simulink model "CL_CC"  (R2015b)
settings: Solver=FixedStepDiscrete  StartTime=0.0  StopTime=final_time  RelTol=1e-3
undefined symbols (not defined in the file): BMSk_stepSize, cell_ocvs_sampling, cell_socs_sampling, cell_temps_sampling, cell_voltages_sampling, charge_cycle, inital_outlet_temperature, initial_cell_ocvs, initial_cell_socs, initial_cell_temps, initial_cell_voltages, initial_pack_current, initial_pack_soc, initial_pack_voltage, initial_vehicle_side_voltage, pack_current_sampling, pack_soc_sampling, pack_voltage_sampling, sigbuilder_block, vehicle_side_voltage_sampling
libraries: simulink x5
(part 2 of 2)

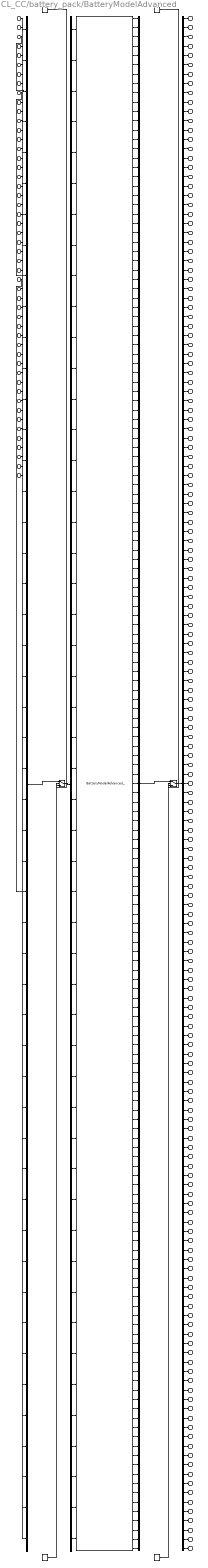
== system CL_CC/battery_pack/BatteryModelAdvanced ==
  cmd_1 : Inport
  cmd_2 : Inport  Port=2
  cmd_3 : Inport  Port=3
  cmd_4 : Inport  Port=4
  cmd_5 : Inport  Port=5
  cmd_6 : Inport  Port=6
  cmd_7 : Inport  Port=7
  cmd_8 : Inport  Port=8
  cmd_9 : Inport  Port=9
  cmd_10 : Inport  Port=10
  cmd_11 : Inport  Port=11
  cmd_12 : Inport  Port=12
  cmd_13 : Inport  Port=13
  cmd_14 : Inport  Port=14
  cmd_15 : Inport  Port=15
  cmd_16 : Inport  Port=16
  cmd_17 : Inport  Port=17
  cmd_18 : Inport  Port=18
  cmd_19 : Inport  Port=19
  cmd_20 : Inport  Port=20
  cmd_21 : Inport  Port=21
  cmd_22 : Inport  Port=22
  cmd_23 : Inport  Port=23
  cmd_24 : Inport  Port=24
  cmd_25 : Inport  Port=25
  cmd_26 : Inport  Port=26
  cmd_27 : Inport  Port=27
  cmd_28 : Inport  Port=28
  cmd_29 : Inport  Port=29
  cmd_30 : Inport  Port=30
  cmd_31 : Inport  Port=31
  cmd_32 : Inport  Port=32
  cmd_33 : Inport  Port=33
  cmd_34 : Inport  Port=34
  cmd_35 : Inport  Port=35
  cmd_36 : Inport  Port=36
  cmd_37 : Inport  Port=37
  cmd_38 : Inport  Port=38
  cmd_39 : Inport  Port=39
  cmd_40 : Inport  Port=40
  main_cc_comd : Inport  Port=41
  pre_cc_cmd : Inport  Port=42
  neg_cc_cmd : Inport  Port=43
  chg_cc_cmd : Inport  Port=44
  fan_cmd : Inport  Port=45
  cabin_temp : Inport  Port=46
  Ichg_max : Inport  Port=47
  Idischg_max : Inport  Port=48
  input_current : Inport  Port=49
  load_type : Inport  Port=50
  Cmd_In : Constant  Value=[1 1 1 1 1 1 1 1 1 1 1 1 1 1 1 1 1 1 1 1 1 1 1 1 1 1 1 1 1 1 1 1 1 1 1 1 1 1 1 1 1 1 1 1 1 1 1 1 1 1]
  Cmd_Out : Constant  Value=[1 1 1 1 1 1 1 1 1 1 1 1 1 1 1 1 1 1 1 1 1 1 1 1 1 1 1 1 1 1 1 1 1 1 1 1 1 1 1 1 1 1 1 1 1 1 1 1 1 1 1 1 1 1 1 1 1 1 1 1 1 1 1 1 1 1 1 1 1 1 1 1 1 1 1 1 1 1 1 1 1 1 1 1 1 1 1 1 1 1 1 1 1 1 1 1 1 1 1 1 1 1 1 1 1 1 1 1 1 1 1 1 1 1 1 1 1 1 1 1 1 1 1 1 1 1 1 1 1 1 1 1 1 1 1 1 1 1 1 1 1 1 1 1 1 1 1 1 1 1 1 1 1 1 1 1 1 1 1 1 1 1 1 1 1]
  Constant_In : Constant  Value=[0 0 0 0 0 0 0 0 0 0 0 0 0 0 0 0 0 0 0 0 0 0 0 0 0 0 0 0 0 0 0 0 0 0 0 0 0 0 0 0 0 0 0 0 0 0 0 0 0 0]
  Constant_Out : Constant  Value=[0 0 0 0 0 0 0 0 0 0 0 0 0 0 0 0 0 0 0 0 0 0 0 0 0 0 0 0 0 0 0 0 0 0 0 0 0 0 0 0 0 0 0 0 0 0 0 0 0 0 0 0 0 0 0 0 0 0 0 0 0 0 0 0 0 0 0 0 0 0 0 0 0 0 0 0 0 0 0 0 0 0 0 0 0 0 0 0 0 0 0 0 0 0 0 0 0 0 0 0 0 0 0 0 0 0 0 0 0 0 0 0 0 0 0 0 0 0 0 0 0 0 0 0 0 0 0 0 0 0 0 0 0 0 0 0 0 0 0 0 0 0 0 0 0 0 0 0 0 0 0 0 0 0 0 0 0 0 0 0 0 0 0 0 0]
  Demux_In : Demux  Outputs=50
  Demux_Out : Demux  Outputs=165
  Mux_In : Mux  Inputs=50
  Mux_Out : Mux  Inputs=165
  S-Function : S-Function  InitFcn=clear BatteryModelAdvanced_  StopFcn=clear BatteryModelAdvanced_  FunctionName=BatteryModelAdvanced_  Parameters="[0.1;0.1;1e-06;0.1;100;0;0;2;0;1;0.001;0;1] ['tcase             ';'dcell             ';'Lcell             ';'Rcell             ';'Dcell2cell        ';'Tair              ';'cell_capacity     ';'initial_sohc      ';'initial_sohr      ';'balance_resistor  ';'Initial_SOC       ';'imbalance_cell_soc';'load_cycle_type   '] [5;2.009e-06;206;37;77;35;8;100;100;1;60;60;1] [] [] ['cycle_name'] ['Drive_Cycles/FTP_72.data']"  SFunctionDeploymentMode=off  EnableBusSupport=off
      mask Display: port_label('output',1,'Cell_Voltage1');port_label('output',2,'Cell_Voltage2');port_label('output',3,'Cell_Voltage3');port_label('output',4,'Cell_Voltage4');port_label('output',5,'Cell_Voltage5');port_label('output',6,'Cell_Voltage6');port_label('output',7,'Cell_Voltage7');port_label('output',8,'Cell_Voltage8');port_label('output',9,'Cell_Voltage9');port_label('output',10,'Cell_Voltage10');port_label('output',11,'Cell_Voltage11');port_label('output',12,'Cell_Voltage12');port_label('output',13,'Cell_Voltage13');port_label('output',14,'Cell_Voltage14');port_label('output',15,'Cell_Voltage15');port_label('output',16,'Cell_Voltage16');port_label('output',17,'Cell_Voltage17');port_label('output',18,'Cell_Voltage18');port_label('output',19,'Cell_Voltage19');port_label('output',20,'Cell_Voltage20');port_label('output',21,'Cell_Voltage21');port_label('output',22,'Cell_Voltage22');port_label('output',23,'Cell_Voltage23');port_label('output',24,'Cell_Voltage24');port_label('output',25,'Cell_Voltage25');port_label('output',26,'Cell_Voltage26');port_label('output',27,'Cell_Voltage27');port_label('output',28,'Cell_Voltage28');port_label('output',29,'Cell_Voltage29');port_label('output',30,'Cell_Voltage30');port_label('output',31,'Cell_Voltage31');port_label('output',32,'Cell_Voltage32');port_label('output',33,'Cell_Voltage33');port_label('output',34,'Cell_Voltage34');port_label('output',35,'Cell_Voltage35');port_label('output',36,'Cell_Voltage36');port_label('output',37,'Cell_Voltage37');port_label('output',38,'Cell_Voltage38');port_label('output',39,'Cell_Voltage39');port_label('output',40,'Cell_Voltage40');port_label('output',41,'Cell_temp1');port_label('output',42,'Cell_temp2');port_label('output',43,'Cell_temp3');port_label('output',44,'Cell_temp4');port_label('output',45,'Cell_temp5');port_label('output',46,'Cell_temp6');port_label('output',47,'Cell_temp7');port_label('output',48,'Cell_temp8');port_label('output',49,'Cell_temp9');port_label('output',50,'Cell_temp10');port_label('output',51,'Cell_temp11');port_label('output',52,'Cell_temp12');port_label('output',53,'Cell_temp13');port_label('output',54,'Cell_temp14');port_label('output',55,'Cell_temp15');port_label('output',56,'Cell_temp16');port_label('output',57,'Cell_temp17');port_label('output',58,'Cell_temp18');port_label('output',59,'Cell_temp19');port_label('output',60,'Cell_temp20');port_label('output',61,'Cell_temp21');port_label('output',62,'Cell_temp22');port_label('output',63,'Cell_temp23');port_label('output',64,'Cell_temp24');port_label('output',65,'Cell_temp25');port_label('output',66,'Cell_temp26');port_label('output',67,'Cell_temp27');port_label('output',68,'Cell_temp28');port_label('output',69,'Cell_temp29');port_label('output',70,'Cell_temp30');port_label('output',71,'Cell_temp31');port_label('output',72,'Cell_temp32');port_label('output',73,'Cell_temp33');port_label('output',74,'Cell_temp34');port_label('output',75,'Cell_temp35');port_label('output',76,'Cell_temp36');port_label('output',77,'Cell_temp37');port_label('output',78,'Cell_temp38');port_label('output',79,'Cell_temp39');port_label('output',80,'Cell_temp40');port_label('output',81,'Cell_soc1');port_label('output',82,'Cell_soc2');port_label('output',83,'Cell_soc3');port_label('output',84,'Cell_soc4');port_label('output',85,'Cell_soc5');port_label('output',86,'Cell_soc6');port_label('output',87,'Cell_soc7');port_label('output',88,'Cell_soc8');port_label('output',89,'Cell_soc9');port_label('output',90,'Cell_soc10');port_label('output',91,'Cell_soc11');port_label('output',92,'Cell_soc12');port_label('output',93,'Cell_soc13');port_label('output',94,'Cell_soc14');port_label('output',95,'Cell_soc15');port_label('output',96,'Cell_soc16');port_label('output',97,'Cell_soc17');port_label('output',98,'Cell_soc18');port_label('output',99,'Cell_soc19');port_label('output',100,'Cell_soc20');port_label('output',101,'Cell_soc21');port_label('output',102,'Cell_soc22');port_label('output',103,'Cell_soc23');port_label('output',104,'Cell_soc24');port_label('output',105,'Cell_soc25');port_label('output',106,'Cell_soc26');port_label('output',107,'Cell_soc27');port_label('output',108,'Cell_soc28');port_label('output',109,'Cell_soc29');port_label('output',110,'Cell_soc30');port_label('output',111,'Cell_soc31');port_label('output',112,'Cell_soc32');port_label('output',113,'Cell_soc33');port_label('output',114,'Cell_soc34');port_label('output',115,'Cell_soc35');port_label('output',116,'Cell_soc36');port_label('output',117,'Cell_soc37');port_label('output',118,'Cell_soc38');port_label('output',119,'Cell_soc39');port_label('output',120,'Cell_soc40');port_label('output',121,'Cell_ocv1');port_label('output',122,'Cell_ocv2');port_label('output',123,'Cell_ocv3');port_label('output',124,'Cell_ocv4');port_label('output',125,'Cell_ocv5');port_label('output',126,'Cell_ocv6');port_label('output',127,'Cell_ocv7');port_label('output',128,'Cell_ocv8');port_label('output',129,'Cell_ocv9');port_label('output',130,'Cell_ocv10');port_label('output',131,'Cell_ocv11');port_label('output',132,'Cell_ocv12');port_label('output',133,'Cell_ocv13');port_label('output',134,'Cell_ocv14');port_label('output',135,'Cell_ocv15');port_label('output',136,'Cell_ocv16');port_label('output',137,'Cell_ocv17');port_label('output',138,'Cell_ocv18');port_label('output',139,'Cell_ocv19');port_label('output',140,'Cell_ocv20');port_label('output',141,'Cell_ocv21');port_label('output',142,'Cell_ocv22');port_label('output',143,'Cell_ocv23');port_label('output',144,'Cell_ocv24');port_label('output',145,'Cell_ocv25');port_label('output',146,'Cell_ocv26');port_label('output',147,'Cell_ocv27');port_label('output',148,'Cell_ocv28');port_label('output',149,'Cell_ocv29');port_label('output',150,'Cell_ocv30');port_label('output',151,'Cell_ocv31');port_label('output',152,'Cell_ocv32');port_label('output',153,'Cell_ocv33');port_label('output',154,'Cell_ocv34');port_label('output',155,'Cell_ocv35');port_label('output',156,'Cell_ocv36');port_label('output',157,'Cell_ocv37');port_label('output',158,'Cell_ocv38');port_label('output',159,'Cell_ocv39');port_label('output',160,'Cell_ocv40');port_label('output',161,'outlet_temperature');port_label('output',162,'pack_voltage');port_label('output',163,'vehicle_side_voltage');port_label('output',164,'pack_current');port_label('output',165,'pack_soc');port_label('input',1,'cmd_1');port_label('input',2,'cmd_2');port_label('input',3,'cmd_3');port_label('input',4,'cmd_4');port_label('input',5,'cmd_5');port_label('input',6,'cmd_6');port_label('input',7,'cmd_7');port_label('input',8,'cmd_8');port_label('input',9,'cmd_9');port_label('input',10,'cmd_10');port_label('input',11,'cmd_11');port_label('input',12,'cmd_12');port_label('input',13,'cmd_13');port_label('input',14,'cmd_14');port_label('input',15,'cmd_15');port_label('input',16,'cmd_16');port_label('input',17,'cmd_17');port_label('input',18,'cmd_18');port_label('input',19,'cmd_19');port_label('input',20,'cmd_20');port_label('input',21,'cmd_21');port_label('input',22,'cmd_22');port_label('input',23,'cmd_23');port_label('input',24,'cmd_24');port_label('input',25,'cmd_25');port_label('input',26,'cmd_26');port_label('input',27,'cmd_27');port_label('input',28,'cmd_28');port_label('input',29,'cmd_29');port_label('input',30,'cmd_30');port_label('input',31,'cmd_31');port_label('input',32,'cmd_32');port_label('input',33,'cmd_33');port_label('input',34,'cmd_34');port_label('input',35,'cmd_35');port_label('input',36,'cmd_36');port_label('input',37,'cmd_37');port_label('input',38,'cmd_38');port_label('input',39,'cmd_39');port_label('input',40,'cmd_40');port_label('input',41,'main_cc_comd');port_label('input',42,'pre_cc_cmd');port_label('input',43,'neg_cc_cmd');port_label('input',44,'chg_cc_cmd');port_label('input',45,'fan_cmd');port_label('input',46,'cabin_temp');port_label('input',47,'Ichg_max');port_label('input',48,'Idischg_max');port_label('input',49,'input_current');port_label('input',50,'load_type');disp('Simcenter Amesim:\n BatteryModelAdvanced_')
  Switch_In : Switch  Threshold=0.5  SaturateOnIntegerOverflow=on  InputSameDT=on
  Switch_Out : Switch  Threshold=0.5  SaturateOnIntegerOverflow=on  InputSameDT=on
  Cell_Voltage1 : Outport
  Cell_Voltage2 : Outport  Port=2
  Cell_Voltage3 : Outport  Port=3
  Cell_Voltage4 : Outport  Port=4
  Cell_Voltage5 : Outport  Port=5
  Cell_Voltage6 : Outport  Port=6
  Cell_Voltage7 : Outport  Port=7
  Cell_Voltage8 : Outport  Port=8
  Cell_Voltage9 : Outport  Port=9
  Cell_Voltage10 : Outport  Port=10
  Cell_Voltage11 : Outport  Port=11
  Cell_Voltage12 : Outport  Port=12
  Cell_Voltage13 : Outport  Port=13
  Cell_Voltage14 : Outport  Port=14
  Cell_Voltage15 : Outport  Port=15
  Cell_Voltage16 : Outport  Port=16
  Cell_Voltage17 : Outport  Port=17
  Cell_Voltage18 : Outport  Port=18
  Cell_Voltage19 : Outport  Port=19
  Cell_Voltage20 : Outport  Port=20
  Cell_Voltage21 : Outport  Port=21
  Cell_Voltage22 : Outport  Port=22
  Cell_Voltage23 : Outport  Port=23
  Cell_Voltage24 : Outport  Port=24
  Cell_Voltage25 : Outport  Port=25
  Cell_Voltage26 : Outport  Port=26
  Cell_Voltage27 : Outport  Port=27
  Cell_Voltage28 : Outport  Port=28
  Cell_Voltage29 : Outport  Port=29
  Cell_Voltage30 : Outport  Port=30
  Cell_Voltage31 : Outport  Port=31
  Cell_Voltage32 : Outport  Port=32
  Cell_Voltage33 : Outport  Port=33
  Cell_Voltage34 : Outport  Port=34
  Cell_Voltage35 : Outport  Port=35
  Cell_Voltage36 : Outport  Port=36
  Cell_Voltage37 : Outport  Port=37
  Cell_Voltage38 : Outport  Port=38
  Cell_Voltage39 : Outport  Port=39
  Cell_Voltage40 : Outport  Port=40
  Cell_temp1 : Outport  Port=41
  Cell_temp2 : Outport  Port=42
  Cell_temp3 : Outport  Port=43
  Cell_temp4 : Outport  Port=44
  Cell_temp5 : Outport  Port=45
  Cell_temp6 : Outport  Port=46
  Cell_temp7 : Outport  Port=47
  Cell_temp8 : Outport  Port=48
  Cell_temp9 : Outport  Port=49
  Cell_temp10 : Outport  Port=50
  Cell_temp11 : Outport  Port=51
  Cell_temp12 : Outport  Port=52
  Cell_temp13 : Outport  Port=53
  Cell_temp14 : Outport  Port=54
  Cell_temp15 : Outport  Port=55
  Cell_temp16 : Outport  Port=56
  Cell_temp17 : Outport  Port=57
  Cell_temp18 : Outport  Port=58
  Cell_temp19 : Outport  Port=59
  Cell_temp20 : Outport  Port=60
  Cell_temp21 : Outport  Port=61
  Cell_temp22 : Outport  Port=62
  Cell_temp23 : Outport  Port=63
  Cell_temp24 : Outport  Port=64
  Cell_temp25 : Outport  Port=65
  Cell_temp26 : Outport  Port=66
  Cell_temp27 : Outport  Port=67
  Cell_temp28 : Outport  Port=68
  Cell_temp29 : Outport  Port=69
  Cell_temp30 : Outport  Port=70
  Cell_temp31 : Outport  Port=71
  Cell_temp32 : Outport  Port=72
  Cell_temp33 : Outport  Port=73
  Cell_temp34 : Outport  Port=74
  Cell_temp35 : Outport  Port=75
  Cell_temp36 : Outport  Port=76
  Cell_temp37 : Outport  Port=77
  Cell_temp38 : Outport  Port=78
  Cell_temp39 : Outport  Port=79
  Cell_temp40 : Outport  Port=80
  Cell_soc1 : Outport  Port=81
  Cell_soc2 : Outport  Port=82
  Cell_soc3 : Outport  Port=83
  Cell_soc4 : Outport  Port=84
  Cell_soc5 : Outport  Port=85
  Cell_soc6 : Outport  Port=86
  Cell_soc7 : Outport  Port=87
  Cell_soc8 : Outport  Port=88
  Cell_soc9 : Outport  Port=89
  Cell_soc10 : Outport  Port=90
  Cell_soc11 : Outport  Port=91
  Cell_soc12 : Outport  Port=92
  Cell_soc13 : Outport  Port=93
  Cell_soc14 : Outport  Port=94
  Cell_soc15 : Outport  Port=95
  Cell_soc16 : Outport  Port=96
  Cell_soc17 : Outport  Port=97
  Cell_soc18 : Outport  Port=98
  Cell_soc19 : Outport  Port=99
  Cell_soc20 : Outport  Port=100
  Cell_soc21 : Outport  Port=101
  Cell_soc22 : Outport  Port=102
  Cell_soc23 : Outport  Port=103
  Cell_soc24 : Outport  Port=104
  Cell_soc25 : Outport  Port=105
  Cell_soc26 : Outport  Port=106
  Cell_soc27 : Outport  Port=107
  Cell_soc28 : Outport  Port=108
  Cell_soc29 : Outport  Port=109
  Cell_soc30 : Outport  Port=110
  Cell_soc31 : Outport  Port=111
  Cell_soc32 : Outport  Port=112
  Cell_soc33 : Outport  Port=113
  Cell_soc34 : Outport  Port=114
  Cell_soc35 : Outport  Port=115
  Cell_soc36 : Outport  Port=116
  Cell_soc37 : Outport  Port=117
  Cell_soc38 : Outport  Port=118
  Cell_soc39 : Outport  Port=119
  Cell_soc40 : Outport  Port=120
  Cell_ocv1 : Outport  Port=121
  Cell_ocv2 : Outport  Port=122
  Cell_ocv3 : Outport  Port=123
  Cell_ocv4 : Outport  Port=124
  Cell_ocv5 : Outport  Port=125
  Cell_ocv6 : Outport  Port=126
  Cell_ocv7 : Outport  Port=127
  Cell_ocv8 : Outport  Port=128
  Cell_ocv9 : Outport  Port=129
  Cell_ocv10 : Outport  Port=130
  Cell_ocv11 : Outport  Port=131
  Cell_ocv12 : Outport  Port=132
  Cell_ocv13 : Outport  Port=133
  Cell_ocv14 : Outport  Port=134
  Cell_ocv15 : Outport  Port=135
  Cell_ocv16 : Outport  Port=136
  Cell_ocv17 : Outport  Port=137
  Cell_ocv18 : Outport  Port=138
  Cell_ocv19 : Outport  Port=139
  Cell_ocv20 : Outport  Port=140
  Cell_ocv21 : Outport  Port=141
  Cell_ocv22 : Outport  Port=142
  Cell_ocv23 : Outport  Port=143
  Cell_ocv24 : Outport  Port=144
  Cell_ocv25 : Outport  Port=145
  Cell_ocv26 : Outport  Port=146
  Cell_ocv27 : Outport  Port=147
  Cell_ocv28 : Outport  Port=148
  Cell_ocv29 : Outport  Port=149
  Cell_ocv30 : Outport  Port=150
  Cell_ocv31 : Outport  Port=151
  Cell_ocv32 : Outport  Port=152
  Cell_ocv33 : Outport  Port=153
  Cell_ocv34 : Outport  Port=154
  Cell_ocv35 : Outport  Port=155
  Cell_ocv36 : Outport  Port=156
  Cell_ocv37 : Outport  Port=157
  Cell_ocv38 : Outport  Port=158
  Cell_ocv39 : Outport  Port=159
  Cell_ocv40 : Outport  Port=160
  outlet_temperature : Outport  Port=161
  pack_voltage : Outport  Port=162
  vehicle_side_voltage : Outport  Port=163
  pack_current : Outport  Port=164
  pack_soc : Outport  Port=165
  wires:
  Mux_In/1 -> Switch_In/1
  Cmd_In/1 -> Switch_In/2
  Constant_In/1 -> Switch_In/3
  Switch_In/1 -> Demux_In/1
  Mux_Out/1 -> Switch_Out/1
  Cmd_Out/1 -> Switch_Out/2
  Constant_Out/1 -> Switch_Out/3
  Switch_Out/1 -> Demux_Out/1
  cmd_1/1 -> Mux_In/1
  Demux_In/1 -> S-Function/1
  cmd_2/1 -> Mux_In/2
  Demux_In/2 -> S-Function/2
  cmd_3/1 -> Mux_In/3
  Demux_In/3 -> S-Function/3
  cmd_4/1 -> Mux_In/4
  Demux_In/4 -> S-Function/4
  cmd_5/1 -> Mux_In/5
  Demux_In/5 -> S-Function/5
  cmd_6/1 -> Mux_In/6
  Demux_In/6 -> S-Function/6
  cmd_7/1 -> Mux_In/7
  Demux_In/7 -> S-Function/7
  cmd_8/1 -> Mux_In/8
  Demux_In/8 -> S-Function/8
  cmd_9/1 -> Mux_In/9
  Demux_In/9 -> S-Function/9
  cmd_10/1 -> Mux_In/10
  Demux_In/10 -> S-Function/10
  cmd_11/1 -> Mux_In/11
  Demux_In/11 -> S-Function/11
  cmd_12/1 -> Mux_In/12
  Demux_In/12 -> S-Function/12
  cmd_13/1 -> Mux_In/13
  Demux_In/13 -> S-Function/13
  cmd_14/1 -> Mux_In/14
  Demux_In/14 -> S-Function/14
  cmd_15/1 -> Mux_In/15
  Demux_In/15 -> S-Function/15
  cmd_16/1 -> Mux_In/16
  Demux_In/16 -> S-Function/16
  cmd_17/1 -> Mux_In/17
  Demux_In/17 -> S-Function/17
  cmd_18/1 -> Mux_In/18
  Demux_In/18 -> S-Function/18
  cmd_19/1 -> Mux_In/19
  Demux_In/19 -> S-Function/19
  cmd_20/1 -> Mux_In/20
  Demux_In/20 -> S-Function/20
  cmd_21/1 -> Mux_In/21
  Demux_In/21 -> S-Function/21
  cmd_22/1 -> Mux_In/22
  Demux_In/22 -> S-Function/22
  cmd_23/1 -> Mux_In/23
  Demux_In/23 -> S-Function/23
  cmd_24/1 -> Mux_In/24
  Demux_In/24 -> S-Function/24
  cmd_25/1 -> Mux_In/25
  Demux_In/25 -> S-Function/25
  cmd_26/1 -> Mux_In/26
  Demux_In/26 -> S-Function/26
  cmd_27/1 -> Mux_In/27
  Demux_In/27 -> S-Function/27
  cmd_28/1 -> Mux_In/28
  Demux_In/28 -> S-Function/28
  cmd_29/1 -> Mux_In/29
  Demux_In/29 -> S-Function/29
  cmd_30/1 -> Mux_In/30
  Demux_In/30 -> S-Function/30
  cmd_31/1 -> Mux_In/31
  Demux_In/31 -> S-Function/31
  cmd_32/1 -> Mux_In/32
  Demux_In/32 -> S-Function/32
  cmd_33/1 -> Mux_In/33
  Demux_In/33 -> S-Function/33
  cmd_34/1 -> Mux_In/34
  Demux_In/34 -> S-Function/34
  cmd_35/1 -> Mux_In/35
  Demux_In/35 -> S-Function/35
  cmd_36/1 -> Mux_In/36
  Demux_In/36 -> S-Function/36
  cmd_37/1 -> Mux_In/37
  Demux_In/37 -> S-Function/37
  cmd_38/1 -> Mux_In/38
  Demux_In/38 -> S-Function/38
  cmd_39/1 -> Mux_In/39
  Demux_In/39 -> S-Function/39
  cmd_40/1 -> Mux_In/40
  Demux_In/40 -> S-Function/40
  main_cc_comd/1 -> Mux_In/41
  Demux_In/41 -> S-Function/41
  pre_cc_cmd/1 -> Mux_In/42
  Demux_In/42 -> S-Function/42
  neg_cc_cmd/1 -> Mux_In/43
  Demux_In/43 -> S-Function/43
  chg_cc_cmd/1 -> Mux_In/44
  Demux_In/44 -> S-Function/44
  fan_cmd/1 -> Mux_In/45
  Demux_In/45 -> S-Function/45
  cabin_temp/1 -> Mux_In/46
  Demux_In/46 -> S-Function/46
  Ichg_max/1 -> Mux_In/47
  Demux_In/47 -> S-Function/47
  Idischg_max/1 -> Mux_In/48
  Demux_In/48 -> S-Function/48
  input_current/1 -> Mux_In/49
  Demux_In/49 -> S-Function/49
  load_type/1 -> Mux_In/50
  Demux_In/50 -> S-Function/50
  Demux_Out/1 -> Cell_Voltage1/1
  S-Function/1 -> Mux_Out/1
  Demux_Out/2 -> Cell_Voltage2/1
  S-Function/2 -> Mux_Out/2
  Demux_Out/3 -> Cell_Voltage3/1
  S-Function/3 -> Mux_Out/3
  Demux_Out/4 -> Cell_Voltage4/1
  S-Function/4 -> Mux_Out/4
  Demux_Out/5 -> Cell_Voltage5/1
  S-Function/5 -> Mux_Out/5
  Demux_Out/6 -> Cell_Voltage6/1
  S-Function/6 -> Mux_Out/6
  Demux_Out/7 -> Cell_Voltage7/1
  S-Function/7 -> Mux_Out/7
  Demux_Out/8 -> Cell_Voltage8/1
  S-Function/8 -> Mux_Out/8
  Demux_Out/9 -> Cell_Voltage9/1
  S-Function/9 -> Mux_Out/9
  Demux_Out/10 -> Cell_Voltage10/1
  S-Function/10 -> Mux_Out/10
  Demux_Out/11 -> Cell_Voltage11/1
  S-Function/11 -> Mux_Out/11
  Demux_Out/12 -> Cell_Voltage12/1
  S-Function/12 -> Mux_Out/12
  Demux_Out/13 -> Cell_Voltage13/1
  S-Function/13 -> Mux_Out/13
  Demux_Out/14 -> Cell_Voltage14/1
  S-Function/14 -> Mux_Out/14
  Demux_Out/15 -> Cell_Voltage15/1
  S-Function/15 -> Mux_Out/15
  Demux_Out/16 -> Cell_Voltage16/1
  S-Function/16 -> Mux_Out/16
  Demux_Out/17 -> Cell_Voltage17/1
  S-Function/17 -> Mux_Out/17
  Demux_Out/18 -> Cell_Voltage18/1
  S-Function/18 -> Mux_Out/18
  Demux_Out/19 -> Cell_Voltage19/1
  S-Function/19 -> Mux_Out/19
  Demux_Out/20 -> Cell_Voltage20/1
  S-Function/20 -> Mux_Out/20
  Demux_Out/21 -> Cell_Voltage21/1
  S-Function/21 -> Mux_Out/21
  Demux_Out/22 -> Cell_Voltage22/1
  S-Function/22 -> Mux_Out/22
  Demux_Out/23 -> Cell_Voltage23/1
  S-Function/23 -> Mux_Out/23
  Demux_Out/24 -> Cell_Voltage24/1
  S-Function/24 -> Mux_Out/24
  Demux_Out/25 -> Cell_Voltage25/1
  S-Function/25 -> Mux_Out/25
  Demux_Out/26 -> Cell_Voltage26/1
  S-Function/26 -> Mux_Out/26
  Demux_Out/27 -> Cell_Voltage27/1
  S-Function/27 -> Mux_Out/27
  Demux_Out/28 -> Cell_Voltage28/1
  S-Function/28 -> Mux_Out/28
  Demux_Out/29 -> Cell_Voltage29/1
  S-Function/29 -> Mux_Out/29
  Demux_Out/30 -> Cell_Voltage30/1
  S-Function/30 -> Mux_Out/30
  Demux_Out/31 -> Cell_Voltage31/1
  S-Function/31 -> Mux_Out/31
  Demux_Out/32 -> Cell_Voltage32/1
  S-Function/32 -> Mux_Out/32
  Demux_Out/33 -> Cell_Voltage33/1
  S-Function/33 -> Mux_Out/33
  Demux_Out/34 -> Cell_Voltage34/1
  S-Function/34 -> Mux_Out/34
  Demux_Out/35 -> Cell_Voltage35/1
  S-Function/35 -> Mux_Out/35
  Demux_Out/36 -> Cell_Voltage36/1
  S-Function/36 -> Mux_Out/36
  Demux_Out/37 -> Cell_Voltage37/1
  S-Function/37 -> Mux_Out/37
  Demux_Out/38 -> Cell_Voltage38/1
  S-Function/38 -> Mux_Out/38
  Demux_Out/39 -> Cell_Voltage39/1
  S-Function/39 -> Mux_Out/39
  Demux_Out/40 -> Cell_Voltage40/1
  S-Function/40 -> Mux_Out/40
  Demux_Out/41 -> Cell_temp1/1
  S-Function/41 -> Mux_Out/41
  Demux_Out/42 -> Cell_temp2/1
  S-Function/42 -> Mux_Out/42
  Demux_Out/43 -> Cell_temp3/1
  S-Function/43 -> Mux_Out/43
  Demux_Out/44 -> Cell_temp4/1
  S-Function/44 -> Mux_Out/44
  Demux_Out/45 -> Cell_temp5/1
  S-Function/45 -> Mux_Out/45
  Demux_Out/46 -> Cell_temp6/1
  S-Function/46 -> Mux_Out/46
  Demux_Out/47 -> Cell_temp7/1
  S-Function/47 -> Mux_Out/47
  Demux_Out/48 -> Cell_temp8/1
  S-Function/48 -> Mux_Out/48
  Demux_Out/49 -> Cell_temp9/1
  S-Function/49 -> Mux_Out/49
  Demux_Out/50 -> Cell_temp10/1
  S-Function/50 -> Mux_Out/50
  Demux_Out/51 -> Cell_temp11/1
  S-Function/51 -> Mux_Out/51
  Demux_Out/52 -> Cell_temp12/1
  S-Function/52 -> Mux_Out/52
  Demux_Out/53 -> Cell_temp13/1
  S-Function/53 -> Mux_Out/53
  Demux_Out/54 -> Cell_temp14/1
  S-Function/54 -> Mux_Out/54
  Demux_Out/55 -> Cell_temp15/1
  S-Function/55 -> Mux_Out/55
  Demux_Out/56 -> Cell_temp16/1
  S-Function/56 -> Mux_Out/56
  Demux_Out/57 -> Cell_temp17/1
  S-Function/57 -> Mux_Out/57
  Demux_Out/58 -> Cell_temp18/1
  S-Function/58 -> Mux_Out/58
  Demux_Out/59 -> Cell_temp19/1
  S-Function/59 -> Mux_Out/59
  Demux_Out/60 -> Cell_temp20/1
  S-Function/60 -> Mux_Out/60
  Demux_Out/61 -> Cell_temp21/1
  S-Function/61 -> Mux_Out/61
  Demux_Out/62 -> Cell_temp22/1
  S-Function/62 -> Mux_Out/62
  Demux_Out/63 -> Cell_temp23/1
  S-Function/63 -> Mux_Out/63
  Demux_Out/64 -> Cell_temp24/1
  S-Function/64 -> Mux_Out/64
  Demux_Out/65 -> Cell_temp25/1
  S-Function/65 -> Mux_Out/65
  Demux_Out/66 -> Cell_temp26/1
  S-Function/66 -> Mux_Out/66
  Demux_Out/67 -> Cell_temp27/1
  S-Function/67 -> Mux_Out/67
  Demux_Out/68 -> Cell_temp28/1
  S-Function/68 -> Mux_Out/68
  Demux_Out/69 -> Cell_temp29/1
  S-Function/69 -> Mux_Out/69
  Demux_Out/70 -> Cell_temp30/1
  S-Function/70 -> Mux_Out/70
  Demux_Out/71 -> Cell_temp31/1
  S-Function/71 -> Mux_Out/71
  Demux_Out/72 -> Cell_temp32/1
  S-Function/72 -> Mux_Out/72
  Demux_Out/73 -> Cell_temp33/1
  S-Function/73 -> Mux_Out/73
  Demux_Out/74 -> Cell_temp34/1
  S-Function/74 -> Mux_Out/74
  Demux_Out/75 -> Cell_temp35/1
  S-Function/75 -> Mux_Out/75
  Demux_Out/76 -> Cell_temp36/1
  S-Function/76 -> Mux_Out/76
  Demux_Out/77 -> Cell_temp37/1
  S-Function/77 -> Mux_Out/77
  Demux_Out/78 -> Cell_temp38/1
  S-Function/78 -> Mux_Out/78
  Demux_Out/79 -> Cell_temp39/1
  S-Function/79 -> Mux_Out/79
  Demux_Out/80 -> Cell_temp40/1
  S-Function/80 -> Mux_Out/80
  Demux_Out/81 -> Cell_soc1/1
  S-Function/81 -> Mux_Out/81
  Demux_Out/82 -> Cell_soc2/1
  S-Function/82 -> Mux_Out/82
  Demux_Out/83 -> Cell_soc3/1
  S-Function/83 -> Mux_Out/83
  Demux_Out/84 -> Cell_soc4/1
  S-Function/84 -> Mux_Out/84
  Demux_Out/85 -> Cell_soc5/1
  S-Function/85 -> Mux_Out/85
  Demux_Out/86 -> Cell_soc6/1
  S-Function/86 -> Mux_Out/86
  Demux_Out/87 -> Cell_soc7/1
  S-Function/87 -> Mux_Out/87
  Demux_Out/88 -> Cell_soc8/1
  S-Function/88 -> Mux_Out/88
  Demux_Out/89 -> Cell_soc9/1
  S-Function/89 -> Mux_Out/89
  Demux_Out/90 -> Cell_soc10/1
  S-Function/90 -> Mux_Out/90
  Demux_Out/91 -> Cell_soc11/1
  S-Function/91 -> Mux_Out/91
  Demux_Out/92 -> Cell_soc12/1
  S-Function/92 -> Mux_Out/92
  Demux_Out/93 -> Cell_soc13/1
  S-Function/93 -> Mux_Out/93
  Demux_Out/94 -> Cell_soc14/1
  S-Function/94 -> Mux_Out/94
  Demux_Out/95 -> Cell_soc15/1
  S-Function/95 -> Mux_Out/95
  Demux_Out/96 -> Cell_soc16/1
  S-Function/96 -> Mux_Out/96
  Demux_Out/97 -> Cell_soc17/1
  S-Function/97 -> Mux_Out/97
  Demux_Out/98 -> Cell_soc18/1
  S-Function/98 -> Mux_Out/98
  Demux_Out/99 -> Cell_soc19/1
  S-Function/99 -> Mux_Out/99
  Demux_Out/100 -> Cell_soc20/1
  S-Function/100 -> Mux_Out/100
  Demux_Out/101 -> Cell_soc21/1
  S-Function/101 -> Mux_Out/101
  Demux_Out/102 -> Cell_soc22/1
  S-Function/102 -> Mux_Out/102
  Demux_Out/103 -> Cell_soc23/1
  S-Function/103 -> Mux_Out/103
  Demux_Out/104 -> Cell_soc24/1
  S-Function/104 -> Mux_Out/104
  Demux_Out/105 -> Cell_soc25/1
  S-Function/105 -> Mux_Out/105
  Demux_Out/106 -> Cell_soc26/1
  S-Function/106 -> Mux_Out/106
  Demux_Out/107 -> Cell_soc27/1
  S-Function/107 -> Mux_Out/107
  Demux_Out/108 -> Cell_soc28/1
  S-Function/108 -> Mux_Out/108
  Demux_Out/109 -> Cell_soc29/1
  S-Function/109 -> Mux_Out/109
  Demux_Out/110 -> Cell_soc30/1
  S-Function/110 -> Mux_Out/110
  Demux_Out/111 -> Cell_soc31/1
  S-Function/111 -> Mux_Out/111
  Demux_Out/112 -> Cell_soc32/1
  S-Function/112 -> Mux_Out/112
  Demux_Out/113 -> Cell_soc33/1
  S-Function/113 -> Mux_Out/113
  Demux_Out/114 -> Cell_soc34/1
  S-Function/114 -> Mux_Out/114
  Demux_Out/115 -> Cell_soc35/1
  S-Function/115 -> Mux_Out/115
  Demux_Out/116 -> Cell_soc36/1
  S-Function/116 -> Mux_Out/116
  Demux_Out/117 -> Cell_soc37/1
  S-Function/117 -> Mux_Out/117
  Demux_Out/118 -> Cell_soc38/1
  S-Function/118 -> Mux_Out/118
  Demux_Out/119 -> Cell_soc39/1
  S-Function/119 -> Mux_Out/119
  Demux_Out/120 -> Cell_soc40/1
  S-Function/120 -> Mux_Out/120
  Demux_Out/121 -> Cell_ocv1/1
  S-Function/121 -> Mux_Out/121
  Demux_Out/122 -> Cell_ocv2/1
  S-Function/122 -> Mux_Out/122
  Demux_Out/123 -> Cell_ocv3/1
  S-Function/123 -> Mux_Out/123
  Demux_Out/124 -> Cell_ocv4/1
  S-Function/124 -> Mux_Out/124
  Demux_Out/125 -> Cell_ocv5/1
  S-Function/125 -> Mux_Out/125
  Demux_Out/126 -> Cell_ocv6/1
  S-Function/126 -> Mux_Out/126
  Demux_Out/127 -> Cell_ocv7/1
  S-Function/127 -> Mux_Out/127
  Demux_Out/128 -> Cell_ocv8/1
  S-Function/128 -> Mux_Out/128
  Demux_Out/129 -> Cell_ocv9/1
  S-Function/129 -> Mux_Out/129
  Demux_Out/130 -> Cell_ocv10/1
  S-Function/130 -> Mux_Out/130
  Demux_Out/131 -> Cell_ocv11/1
  S-Function/131 -> Mux_Out/131
  Demux_Out/132 -> Cell_ocv12/1
  S-Function/132 -> Mux_Out/132
  Demux_Out/133 -> Cell_ocv13/1
  S-Function/133 -> Mux_Out/133
  Demux_Out/134 -> Cell_ocv14/1
  S-Function/134 -> Mux_Out/134
  Demux_Out/135 -> Cell_ocv15/1
  S-Function/135 -> Mux_Out/135
  Demux_Out/136 -> Cell_ocv16/1
  S-Function/136 -> Mux_Out/136
  Demux_Out/137 -> Cell_ocv17/1
  S-Function/137 -> Mux_Out/137
  Demux_Out/138 -> Cell_ocv18/1
  S-Function/138 -> Mux_Out/138
  Demux_Out/139 -> Cell_ocv19/1
  S-Function/139 -> Mux_Out/139
  Demux_Out/140 -> Cell_ocv20/1
  S-Function/140 -> Mux_Out/140
  Demux_Out/141 -> Cell_ocv21/1
  S-Function/141 -> Mux_Out/141
  Demux_Out/142 -> Cell_ocv22/1
  S-Function/142 -> Mux_Out/142
  Demux_Out/143 -> Cell_ocv23/1
  S-Function/143 -> Mux_Out/143
  Demux_Out/144 -> Cell_ocv24/1
  S-Function/144 -> Mux_Out/144
  Demux_Out/145 -> Cell_ocv25/1
  S-Function/145 -> Mux_Out/145
  Demux_Out/146 -> Cell_ocv26/1
  S-Function/146 -> Mux_Out/146
  Demux_Out/147 -> Cell_ocv27/1
  S-Function/147 -> Mux_Out/147
  Demux_Out/148 -> Cell_ocv28/1
  S-Function/148 -> Mux_Out/148
  Demux_Out/149 -> Cell_ocv29/1
  S-Function/149 -> Mux_Out/149
  Demux_Out/150 -> Cell_ocv30/1
  S-Function/150 -> Mux_Out/150
  Demux_Out/151 -> Cell_ocv31/1
  S-Function/151 -> Mux_Out/151
  Demux_Out/152 -> Cell_ocv32/1
  S-Function/152 -> Mux_Out/152
  Demux_Out/153 -> Cell_ocv33/1
  S-Function/153 -> Mux_Out/153
  Demux_Out/154 -> Cell_ocv34/1
  S-Function/154 -> Mux_Out/154
  Demux_Out/155 -> Cell_ocv35/1
  S-Function/155 -> Mux_Out/155
  Demux_Out/156 -> Cell_ocv36/1
  S-Function/156 -> Mux_Out/156
  Demux_Out/157 -> Cell_ocv37/1
  S-Function/157 -> Mux_Out/157
  Demux_Out/158 -> Cell_ocv38/1
  S-Function/158 -> Mux_Out/158
  Demux_Out/159 -> Cell_ocv39/1
  S-Function/159 -> Mux_Out/159
  Demux_Out/160 -> Cell_ocv40/1
  S-Function/160 -> Mux_Out/160
  Demux_Out/161 -> outlet_temperature/1
  S-Function/161 -> Mux_Out/161
  Demux_Out/162 -> pack_voltage/1
  S-Function/162 -> Mux_Out/162
  Demux_Out/163 -> vehicle_side_voltage/1
  S-Function/163 -> Mux_Out/163
  Demux_Out/164 -> pack_current/1
  S-Function/164 -> Mux_Out/164
  Demux_Out/165 -> pack_soc/1
  S-Function/165 -> Mux_Out/165

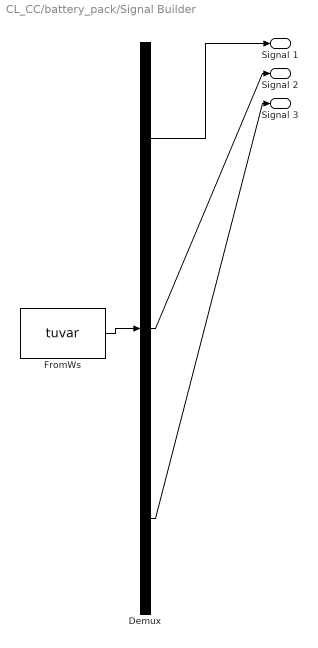
== system CL_CC/battery_pack/Signal Builder ==
  Demux : Demux  Tag=STV Demux  Outputs=3
  FromWs : FromWorkspace  Tag=STV FromWs  VariableName=tuvar  SampleTime=0
      SigBuilderData=|
      | common.afterFinalStr = 'Extrapolate'
      | common.sampleTime = 0
      | dataSet.timeRange = [0 10]
      | dataSet.name = 'Group 1'
      | sbobj.Groups.Name = 'Group 1'
      | sbobj.Groups.Signals(1).Name = 'Signal 1'
      | sbobj.Groups.Signals(1).XData = [0 3 3 3.99 3.99 10]
      | sbobj.Groups.Signals(1).YData = [0 0 1 1 0 0]
      | sbobj.Groups.Signals(2).Name = 'Signal 2'
      | sbobj.Groups.Signals(2).XData = [0 3.76 3.76 10]
      | sbobj.Groups.Signals(2).YData = [0 0 1 1]
      | sbobj.Groups.Signals(3).Name = 'Signal 3'
      | sbobj.Groups.Signals(3).XData = [0 3 3 10]
      | sbobj.Groups.Signals(3).YData = [0 0 1 1]
  Signal 1 : Outport  Tag=STV Outport
  Signal 2 : Outport  Tag=STV Outport  Port=2
  Signal 3 : Outport  Tag=STV Outport  Port=3
  wires:
  Demux/1 -> Signal 1/1
  FromWs/1 -> Demux/1
  Demux/2 -> Signal 2/1
  Demux/3 -> Signal 3/1

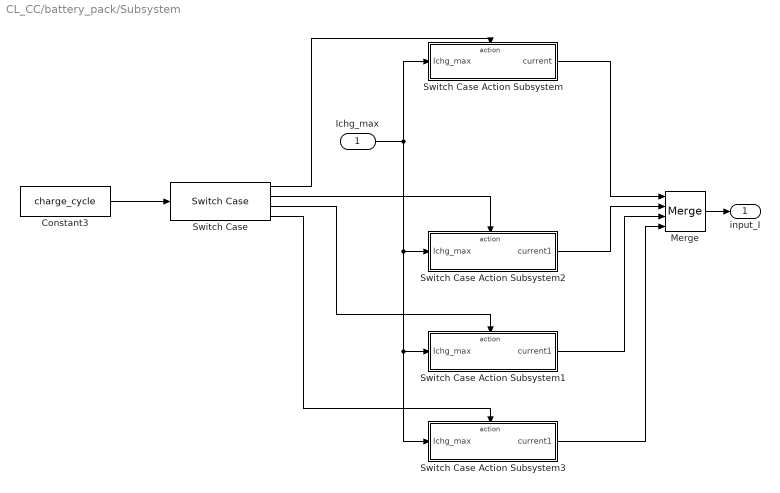
== system CL_CC/battery_pack/Subsystem ==
  Ichg_max : Inport
  Constant3 : Constant  Value=charge_cycle  SampleTime=BMSk_stepSize
  Merge : Merge  Inputs=4
  Switch Case : SwitchCase  CaseConditions={1,2,3,4}  ShowDefaultCase=off
  Switch Case Action Subsystem : Subsystem  TreatAsAtomicUnit=on
  Switch Case Action Subsystem1 : Subsystem  TreatAsAtomicUnit=on
  Switch Case Action Subsystem2 : Subsystem  TreatAsAtomicUnit=on
  Switch Case Action Subsystem3 : Subsystem  TreatAsAtomicUnit=on
  input_I : Outport
  wires:
  Constant3/1 -> Switch Case/1
  Merge/1 -> input_I/1
  Switch Case/1 -> Switch Case Action Subsystem/Action
  Ichg_max/1 -> Switch Case Action Subsystem3/1(Ichg_max), Switch Case Action Subsystem1/1(Ichg_max), Switch Case Action Subsystem2/1(Ichg_max), Switch Case Action Subsystem/1(Ichg_max)
  Switch Case Action Subsystem/1(current) -> Merge/1
  Switch Case Action Subsystem2/1(current1) -> Merge/2
  Switch Case Action Subsystem1/1(current1) -> Merge/3
  Switch Case/2 -> Switch Case Action Subsystem2/Action
  Switch Case/3 -> Switch Case Action Subsystem1/Action
  Switch Case Action Subsystem3/1(current1) -> Merge/4
  Switch Case/4 -> Switch Case Action Subsystem3/Action

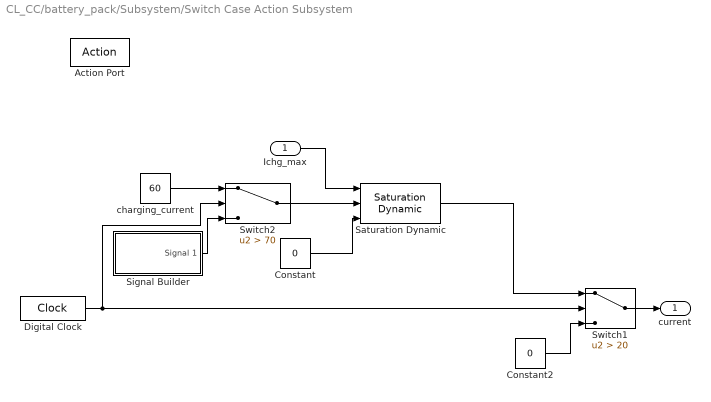
== system CL_CC/battery_pack/Subsystem/Switch Case Action Subsystem ==
  Ichg_max : Inport
  Action Port : ActionPort  ActionType=case
  Constant : Constant  Value=0  SampleTime=BMSk_stepSize
  Constant2 : Constant  Value=0  SampleTime=BMSk_stepSize
  Digital Clock : DigitalClock  SampleTime=BMSk_stepSize
  Saturation Dynamic : simulink/Discontinuities/Saturation Dynamic  OutMin=[]  OutMax=[]  OutDataTypeStr=Inherit: Same as second input  OutDataType=fixdt(1, 16)  OutScaling=2^-10  DoSatur=off
  Signal Builder : Subsystem  Tag=STV Subsys  LoadFcn=sigbuilder_block('load');  StartFcn=sigbuilder_block('start');  StopFcn=sigbuilder_block('stop');  ClipboardFcn=sigbuilder_block('clipboard');  mask(Sigbuilder block){}
      mask help: Simulink:masks:SigbuilderBlock_MD
      mask init:
      | if ~strcmp(get_param(bdroot(gcbh),'SimulationStatus'),'stopped') tuvar = sigbuilder_block('maskInit'); end
      settings: CopyFcn=sigbuilder_block('copy');  DeleteFcn=sigbuilder_block('delete');  ModelCloseFcn=sigbuilder_block('modelClose');  PreSaveFcn=sigbuilder_block('preSave');  PauseFcn=sigbuilder_block('pause');  ContinueFcn=sigbuilder_block('continue');  NameChangeFcn=sigbuilder_block('namechange');  OpenFcn=sigbuilder_block('open',[445.8 137.4 550.8 400.2 ]);  CloseFcn=sigbuilder_block('close');
      mask Display: plot(0, 0, 100, 100,[2, 2, 32, 32, 2], [68, 8, 8, 68, 68],[32, 2], [38, 38], [32, 19, 2],[53, 60, 44], [32, 17, 17, 2],[16, 16, 31, 31]);txt = getActiveGroup(gcbh);text(2, 100, txt,'verticalAlignment', 'top');
  Switch1 : Switch  Criteria=u2 > Threshold  Threshold=20
  Switch2 : Switch  Criteria=u2 > Threshold  Threshold=70
  charging_current : Constant  Value=60  SampleTime=BMSk_stepSize
  current : Outport
  wires:
  Constant/1 -> Saturation Dynamic/3
  Saturation Dynamic/1 -> Switch1/1
  Constant2/1 -> Switch1/3
  charging_current/1 -> Switch2/1
  Signal Builder/1(Signal 1) -> Switch2/3
  Switch2/1 -> Saturation Dynamic/2
  Ichg_max/1 -> Saturation Dynamic/1
  Digital Clock/1 -> Switch2/2, Switch1/2
  Switch1/1 -> current/1

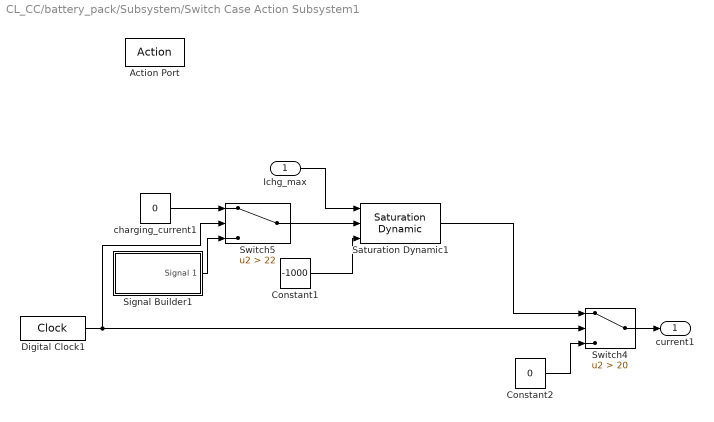
== system CL_CC/battery_pack/Subsystem/Switch Case Action Subsystem1 ==
  Ichg_max : Inport
  Action Port : ActionPort  ActionType=case
  Constant1 : Constant  Value=-1000  SampleTime=BMSk_stepSize
  Constant2 : Constant  Value=0  SampleTime=BMSk_stepSize
  Digital Clock1 : DigitalClock  SampleTime=BMSk_stepSize
  Saturation Dynamic1 : simulink/Discontinuities/Saturation Dynamic  OutMin=[]  OutMax=[]  OutDataTypeStr=Inherit: Same as second input  OutDataType=fixdt(1, 16)  OutScaling=2^-10  DoSatur=off
  Signal Builder1 : Subsystem  Tag=STV Subsys  LoadFcn=sigbuilder_block('load');  StartFcn=sigbuilder_block('start');  StopFcn=sigbuilder_block('stop');  ClipboardFcn=sigbuilder_block('clipboard');  mask(Sigbuilder block){}
      mask help: Simulink:masks:SigbuilderBlock_MD
      mask init:
      | if ~strcmp(get_param(bdroot(gcbh),'SimulationStatus'),'stopped') tuvar = sigbuilder_block('maskInit'); end
      settings: CopyFcn=sigbuilder_block('copy');  DeleteFcn=sigbuilder_block('delete');  ModelCloseFcn=sigbuilder_block('modelClose');  PreSaveFcn=sigbuilder_block('preSave');  PauseFcn=sigbuilder_block('pause');  ContinueFcn=sigbuilder_block('continue');  NameChangeFcn=sigbuilder_block('namechange');  OpenFcn=sigbuilder_block('open',[445.8 137.4 550.8 400.2 ]);  CloseFcn=sigbuilder_block('close');
      mask Display: plot(0, 0, 100, 100,[2, 2, 32, 32, 2], [68, 8, 8, 68, 68],[32, 2], [38, 38], [32, 19, 2],[53, 60, 44], [32, 17, 17, 2],[16, 16, 31, 31]);txt = getActiveGroup(gcbh);text(2, 100, txt,'verticalAlignment', 'top');
  Switch4 : Switch  Criteria=u2 > Threshold  Threshold=20
  Switch5 : Switch  Criteria=u2 > Threshold  Threshold=22
  charging_current1 : Constant  Value=0  SampleTime=BMSk_stepSize
  current1 : Outport
  wires:
  Switch4/1 -> current1/1
  Digital Clock1/1 -> Switch4/2, Switch5/2
  Ichg_max/1 -> Saturation Dynamic1/1
  Switch5/1 -> Saturation Dynamic1/2
  Signal Builder1/1(Signal 1) -> Switch5/3
  charging_current1/1 -> Switch5/1
  Constant2/1 -> Switch4/3
  Saturation Dynamic1/1 -> Switch4/1
  Constant1/1 -> Saturation Dynamic1/3

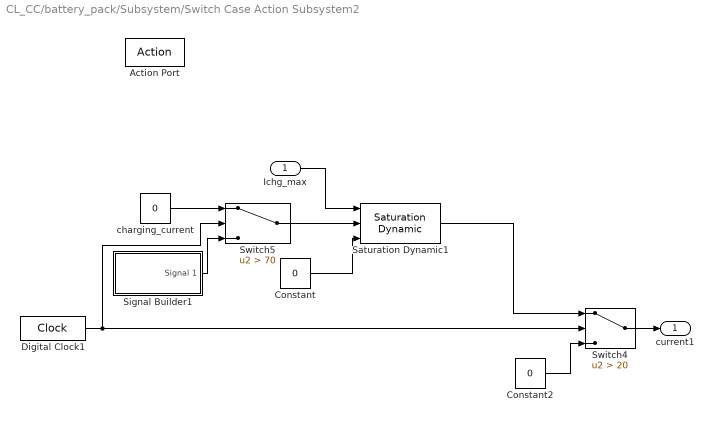
== system CL_CC/battery_pack/Subsystem/Switch Case Action Subsystem2 ==
  Ichg_max : Inport
  Action Port : ActionPort  ActionType=case
  Constant : Constant  Value=0  SampleTime=BMSk_stepSize
  Constant2 : Constant  Value=0  SampleTime=BMSk_stepSize
  Digital Clock1 : DigitalClock  SampleTime=BMSk_stepSize
  Saturation Dynamic1 : simulink/Discontinuities/Saturation Dynamic  OutMin=[]  OutMax=[]  OutDataTypeStr=Inherit: Same as second input  OutDataType=fixdt(1, 16)  OutScaling=2^-10  DoSatur=off
  Signal Builder1 : Subsystem  Tag=STV Subsys  LoadFcn=sigbuilder_block('load');  StartFcn=sigbuilder_block('start');  StopFcn=sigbuilder_block('stop');  ClipboardFcn=sigbuilder_block('clipboard');  mask(Sigbuilder block){}
      mask help: Simulink:masks:SigbuilderBlock_MD
      mask init:
      | if ~strcmp(get_param(bdroot(gcbh),'SimulationStatus'),'stopped') tuvar = sigbuilder_block('maskInit'); end
      settings: CopyFcn=sigbuilder_block('copy');  DeleteFcn=sigbuilder_block('delete');  ModelCloseFcn=sigbuilder_block('modelClose');  PreSaveFcn=sigbuilder_block('preSave');  PauseFcn=sigbuilder_block('pause');  ContinueFcn=sigbuilder_block('continue');  NameChangeFcn=sigbuilder_block('namechange');  OpenFcn=sigbuilder_block('open',[445.8 137.4 550.8 400.2 ]);  CloseFcn=sigbuilder_block('close');
      mask Display: plot(0, 0, 100, 100,[2, 2, 32, 32, 2], [68, 8, 8, 68, 68],[32, 2], [38, 38], [32, 19, 2],[53, 60, 44], [32, 17, 17, 2],[16, 16, 31, 31]);txt = getActiveGroup(gcbh);text(2, 100, txt,'verticalAlignment', 'top');
  Switch4 : Switch  Criteria=u2 > Threshold  Threshold=20
  Switch5 : Switch  Criteria=u2 > Threshold  Threshold=70
  charging_current : Constant  Value=0  SampleTime=BMSk_stepSize
  current1 : Outport
  wires:
  Constant/1 -> Saturation Dynamic1/3
  Saturation Dynamic1/1 -> Switch4/1
  Constant2/1 -> Switch4/3
  charging_current/1 -> Switch5/1
  Signal Builder1/1(Signal 1) -> Switch5/3
  Switch5/1 -> Saturation Dynamic1/2
  Ichg_max/1 -> Saturation Dynamic1/1
  Digital Clock1/1 -> Switch5/2, Switch4/2
  Switch4/1 -> current1/1

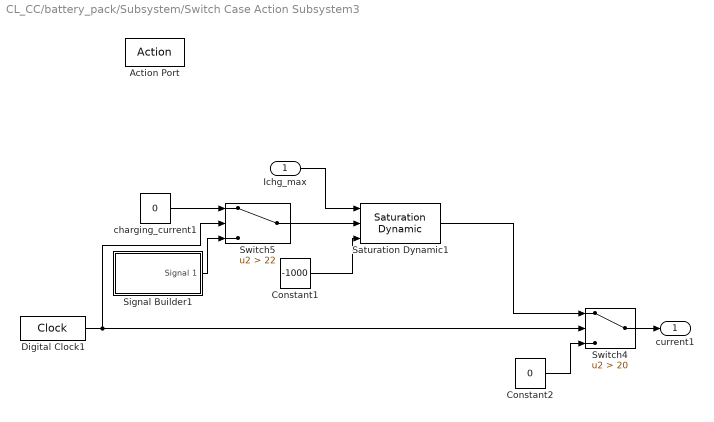
== system CL_CC/battery_pack/Subsystem/Switch Case Action Subsystem3 ==
  Ichg_max : Inport
  Action Port : ActionPort  ActionType=case
  Constant1 : Constant  Value=-1000  SampleTime=BMSk_stepSize
  Constant2 : Constant  Value=0  SampleTime=BMSk_stepSize
  Digital Clock1 : DigitalClock  SampleTime=BMSk_stepSize
  Saturation Dynamic1 : simulink/Discontinuities/Saturation Dynamic  OutMin=[]  OutMax=[]  OutDataTypeStr=Inherit: Same as second input  OutDataType=fixdt(1, 16)  OutScaling=2^-10  DoSatur=off
  Signal Builder1 : Subsystem  Tag=STV Subsys  LoadFcn=sigbuilder_block('load');  StartFcn=sigbuilder_block('start');  StopFcn=sigbuilder_block('stop');  ClipboardFcn=sigbuilder_block('clipboard');  mask(Sigbuilder block){}
      mask help: Simulink:masks:SigbuilderBlock_MD
      mask init:
      | if ~strcmp(get_param(bdroot(gcbh),'SimulationStatus'),'stopped') tuvar = sigbuilder_block('maskInit'); end
      settings: CopyFcn=sigbuilder_block('copy');  DeleteFcn=sigbuilder_block('delete');  ModelCloseFcn=sigbuilder_block('modelClose');  PreSaveFcn=sigbuilder_block('preSave');  PauseFcn=sigbuilder_block('pause');  ContinueFcn=sigbuilder_block('continue');  NameChangeFcn=sigbuilder_block('namechange');  OpenFcn=sigbuilder_block('open',[445.8 137.4 550.8 400.2 ]);  CloseFcn=sigbuilder_block('close');
      mask Display: plot(0, 0, 100, 100,[2, 2, 32, 32, 2], [68, 8, 8, 68, 68],[32, 2], [38, 38], [32, 19, 2],[53, 60, 44], [32, 17, 17, 2],[16, 16, 31, 31]);txt = getActiveGroup(gcbh);text(2, 100, txt,'verticalAlignment', 'top');
  Switch4 : Switch  Criteria=u2 > Threshold  Threshold=20
  Switch5 : Switch  Criteria=u2 > Threshold  Threshold=22
  charging_current1 : Constant  Value=0  SampleTime=BMSk_stepSize
  current1 : Outport
  wires:
  Constant1/1 -> Saturation Dynamic1/3
  Saturation Dynamic1/1 -> Switch4/1
  Constant2/1 -> Switch4/3
  charging_current1/1 -> Switch5/1
  Signal Builder1/1(Signal 1) -> Switch5/3
  Switch5/1 -> Saturation Dynamic1/2
  Ichg_max/1 -> Saturation Dynamic1/1
  Digital Clock1/1 -> Switch5/2, Switch4/2
  Switch4/1 -> current1/1

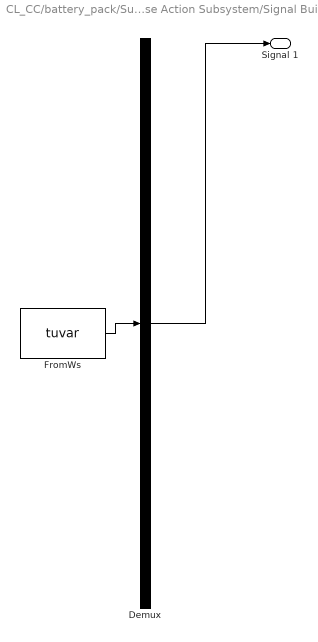
== system CL_CC/battery_pack/Subsystem/Switch Case Action Subsystem/Signal Builder ==
  Demux : Demux  Tag=STV Demux  Outputs=1
  FromWs : FromWorkspace  Tag=STV FromWs  VariableName=tuvar  SampleTime=BMSk_stepSize
      SigBuilderData=|
      | common.afterFinalStr = 'Extrapolate'
      | common.sampleTime = 'BMSk_stepSize'
      | dataSet.timeRange = [20 70]
      | dataSet.name = 'Group 1'
      | sbobj.Groups.Name = 'Group 1'
      | sbobj.Groups.Signals.Name = 'Signal 1'
      | sbobj.Groups.Signals.XData = [20 70]
      | sbobj.Groups.Signals.YData = [40 60]
      | sbobj.Groups.TimeRange = [20 70]
  Signal 1 : Outport  Tag=STV Outport
  wires:
  Demux/1 -> Signal 1/1
  FromWs/1 -> Demux/1

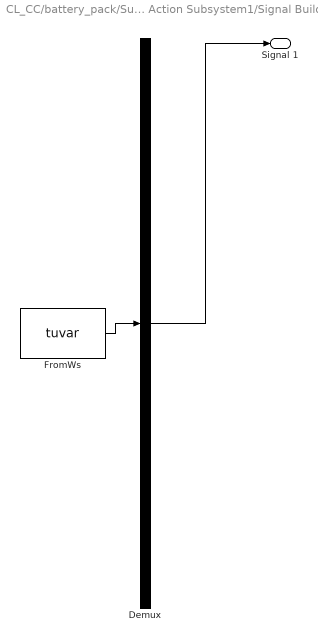
== system CL_CC/battery_pack/Subsystem/Switch Case Action Subsystem1/Signal Builder1 ==
  Demux : Demux  Tag=STV Demux  Outputs=1
  FromWs : FromWorkspace  Tag=STV FromWs  VariableName=tuvar  SampleTime=BMSk_stepSize
      SigBuilderData=|
      | common.afterFinalStr = 'Extrapolate'
      | common.sampleTime = 'BMSk_stepSize'
      | dataSet.timeRange = [20 22]
      | dataSet.name = 'Group 1'
      | sbobj.Groups.Name = 'Group 1'
      | sbobj.Groups.Signals.Name = 'Signal 1'
      | sbobj.Groups.Signals.XData = [20 22]
      | sbobj.Groups.Signals.YData = [-40 -500]
      | sbobj.Groups.TimeRange = [20 22]
  Signal 1 : Outport  Tag=STV Outport
  wires:
  FromWs/1 -> Demux/1
  Demux/1 -> Signal 1/1

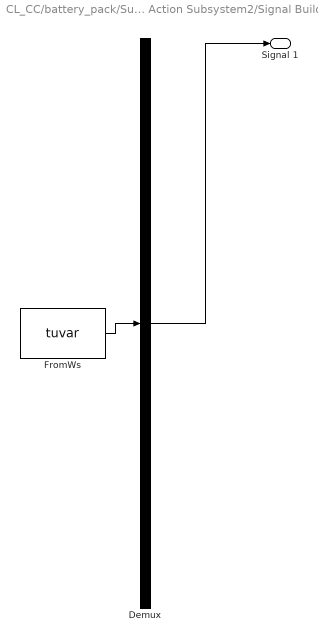
== system CL_CC/battery_pack/Subsystem/Switch Case Action Subsystem2/Signal Builder1 ==
  Demux : Demux  Tag=STV Demux  Outputs=1
  FromWs : FromWorkspace  Tag=STV FromWs  VariableName=tuvar  SampleTime=BMSk_stepSize
      SigBuilderData=|
      | common.afterFinalStr = 'Extrapolate'
      | common.sampleTime = 'BMSk_stepSize'
      | dataSet.timeRange = [20 70]
      | dataSet.name = 'Group 1'
      | sbobj.Groups.Name = 'Group 1'
      | sbobj.Groups.Signals.Name = 'Signal 1'
      | sbobj.Groups.Signals.XData = [20 70]
      | sbobj.Groups.Signals.YData = [40 60]
      | sbobj.Groups.TimeRange = [20 70]
  Signal 1 : Outport  Tag=STV Outport
  wires:
  Demux/1 -> Signal 1/1
  FromWs/1 -> Demux/1

== system CL_CC/battery_pack/Subsystem/Switch Case Action Subsystem3/Signal Builder1 ==
  Demux : Demux  Tag=STV Demux  Outputs=1
  FromWs : FromWorkspace  Tag=STV FromWs  VariableName=tuvar  SampleTime=BMSk_stepSize
      SigBuilderData=|
      | common.afterFinalStr = 'Extrapolate'
      | common.sampleTime = 'BMSk_stepSize'
      | dataSet.timeRange = [20 22]
      | dataSet.name = 'Group 1'
      | sbobj.Groups.Name = 'Group 1'
      | sbobj.Groups.Signals.Name = 'Signal 1'
      | sbobj.Groups.Signals.XData = [20 22]
      | sbobj.Groups.Signals.YData = [40 500]
      | sbobj.Groups.TimeRange = [20 22]
  Signal 1 : Outport  Tag=STV Outport
  wires:
  Demux/1 -> Signal 1/1
  FromWs/1 -> Demux/1
